simulink subsystem "DCEquivalentMaxon_ECX_Speed_16L_48V_40W"  (R2026a)
settings: Solver=VariableStepAuto
libraries: ee_lib x1, fl_lib x1
settings Model: DataDictionary=neck_mk3.sldd  EnableAccessToBaseWorkspace=off  Creator=upattacini  LastModifiedBy=upattacini

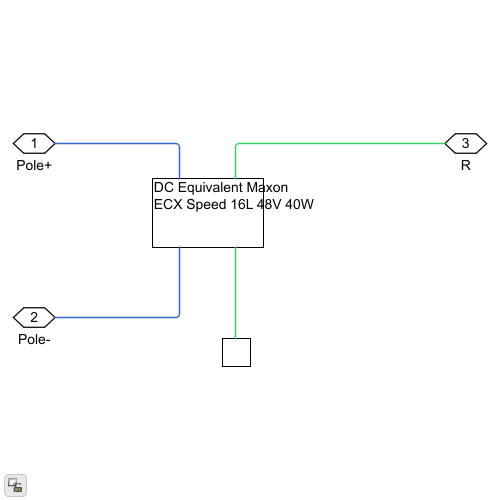
[thumbnail: Simulink's stored preview of the top-level diagram]
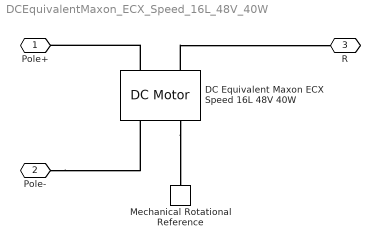
== system DCEquivalentMaxon_ECX_Speed_16L_48V_40W ==
  DC Equivalent Maxon ECX Speed 16L 48V 40W : ee_lib/Electromechanical/Brushed Motors/DC Motor  field_option=ee.enum.field_option.pm  Rf=100 Ohm  Lf=1 H  Laf=0.15 H  If0=0 A  parameterization=ee.enum.dcparam_option.circuit_param  Ra=2.45 / 2 Ohm  La=0.149 mH  emf_or_torque=ee.enum.emf_or_torque.ki  Kv=0.072e-3 V/rpm  Ki=9.31 * sqrt(3/2) mN*m/A  T_stall=0.24e-3 N*m  w_max=19100 rpm  w_rated=15000 rpm  P_rated=0.08 W  V_rated=48 V  lam_param=ee.enum.lam_param.current  i_noload=134 mA  V_i_noload=48 V  J=0.997 cm^2*g  lam=0.00003535461 N*m*s/rad  speed0=0 rpm  alpha=3.93e-3 1/K  Tmeas=25 degC  thermal_mass=100 J/K  initial_temperature=25 degC
  Mechanical Rotational Reference : fl_lib/Mechanical/Rotational Elements/Mechanical Rotational Reference
  Pole+ : PMIOPort  Side=Left
  Pole- : PMIOPort  Port=2  Side=Left
  R : PMIOPort  Port=3  Side=Right
  connections:
  DC Equivalent Maxon ECX Speed 16L 48V 40W/RConn2 -- Mechanical Rotational Reference/LConn1
  DC Equivalent Maxon ECX Speed 16L 48V 40W/LConn1 -- Pole+/RConn1
  DC Equivalent Maxon ECX Speed 16L 48V 40W/LConn2 -- R/RConn1
  Pole-/RConn1 -- DC Equivalent Maxon ECX Speed 16L 48V 40W/RConn1
